simulink model "EXPT_7_7"  (R2019a)
settings: Solver=VariableStepAuto  StartTime=0.0  StopTime=10.0  RelTol=1e-3
undefined symbols (not defined in the file or in its folder): strel
libraries: visionmorphops x4, visionconversions x4, visionsources x1
settings Model: Creator=91977  LastModifiedBy=91977

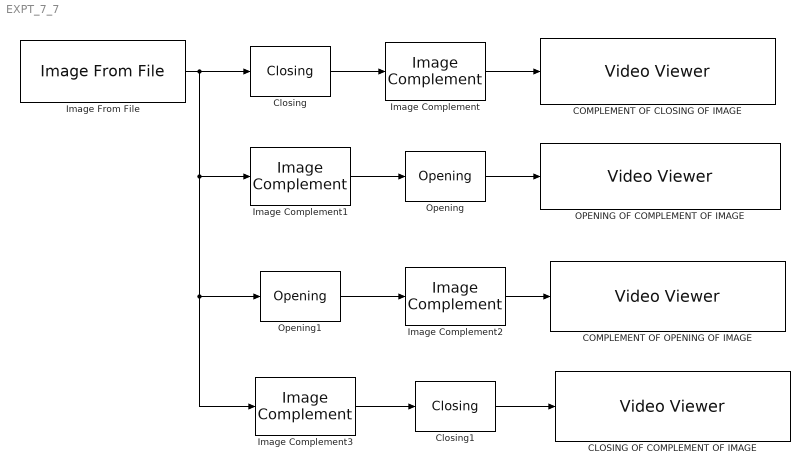
== system EXPT_7_7 ==
  CLOSING OF COMPLEMENT OF IMAGE : VideoViewer  FigPos=[320.2 414.8 417.6 304]
  COMPLEMENT OF CLOSING OF IMAGE : VideoViewer  FigPos=[739.4 826 417.6 304]
  COMPLEMENT OF OPENING OF IMAGE : VideoViewer  FigPos=[739.4 415.6 417.6 304]
  Closing : visionmorphops/Closing  nhoodsrc=Specify via dialog  strel=strel('line',5,45)
      settings: SourceProductName=Computer Vision Toolbox  SourceProductBaseCode=VP
  Closing1 : visionmorphops/Closing  nhoodsrc=Specify via dialog  strel=strel('line',5,45)
      settings: SourceProductName=Computer Vision Toolbox  SourceProductBaseCode=VP
  Image Complement{,1..3} (4 alike) : visionconversions/Image Complement
      settings: SourceProductName=Computer Vision Toolbox  SourceProductBaseCode=VP
  Image From File : visionsources/Image From File  Tag=vipblks_nd  FileName=circles.png  Ts=inf  imagePorts=One multidimensional signal  OutPortLabels=R|G|B  ImageDataType=Inherit from input image  sdImageDataType=uint(8)  Signed=on  WordLength=16  FractionLengthMode=User-defined  FractionLength=15
      settings: SourceProductName=Computer Vision Toolbox
  OPENING OF COMPLEMENT OF IMAGE : VideoViewer  FigPos=[321.8 825.2 417.6 304]
  Opening : visionmorphops/Opening  nhoodsrc=Specify via dialog  strel=strel('disk',5)
      settings: SourceProductName=Computer Vision Toolbox  SourceProductBaseCode=VP
  Opening1 : visionmorphops/Opening  nhoodsrc=Specify via dialog  strel=strel('disk',5)
      settings: SourceProductName=Computer Vision Toolbox  SourceProductBaseCode=VP
  wires:
  Closing1/1 -> CLOSING OF COMPLEMENT OF IMAGE/1
  Image Complement2/1 -> COMPLEMENT OF OPENING OF IMAGE/1
  Opening/1 -> OPENING OF COMPLEMENT OF IMAGE/1
  Image Complement/1 -> COMPLEMENT OF CLOSING OF IMAGE/1
  Closing/1 -> Image Complement/1
  Image Complement1/1 -> Opening/1
  Opening1/1 -> Image Complement2/1
  Image Complement3/1 -> Closing1/1
  Image From File/1 -> Image Complement1/1, Opening1/1, Image Complement3/1, Closing/1
